simulink model "Sri_Lanka_S_FINAL"  (R2024a)
settings: Solver=VariableStepAuto  StartTime=0.0  StopTime=600  RelTol=1e-3
values from neighbouring files (symbols this model uses):
  BRO_R_P = 0.05    [FUtureGridSL.m]    (also in Sri_Lanka_FINAL.m)
  BRO_R_T = 0.38    [FUtureGridSL.m]    (also in Sri_Lanka_FINAL.m)
  BRO_T_G = 0.2    [FUtureGridSL.m]    (also in Sri_Lanka_FINAL.m)
  BRO_T_R = 5.0    (= 5)    [FUtureGridSL.m]    (also in Sri_Lanka_FINAL.m)
  BRO_T_W = 1.0    (= 1)    [FUtureGridSL.m]    (also in Sri_Lanka_FINAL.m)
  BRO_Unit_S_nom = 17.5e6    (= 17500000)    [FUtureGridSL.m]    (also in Sri_Lanka_FINAL.m)
  BWT_R_P = 0.05    [FUtureGridSL.m]    (also in Sri_Lanka.m; Sri_Lanka_FINAL.m)
  BWT_R_T = 0.38    [FUtureGridSL.m]    (also in Sri_Lanka.m; Sri_Lanka_FINAL.m)
  BWT_T_R = 5.0    (= 5)    [FUtureGridSL.m]    (also in Sri_Lanka.m; Sri_Lanka_FINAL.m)
  BWT_T_W = 1.5    [FUtureGridSL.m]    (also in Sri_Lanka.m; Sri_Lanka_FINAL.m)
  BWT_Unit_S_nom = 40e6    (= 40000000)    [FUtureGridSL.m]    (also in Sri_Lanka.m; Sri_Lanka_FINAL.m)
  CAN_R_P = 0.05    [FUtureGridSL.m]    (also in Sri_Lanka_FINAL.m)
  CAN_R_T = 0.38    [FUtureGridSL.m]    (also in Sri_Lanka_FINAL.m)
  CAN_T_G = 0.2    [FUtureGridSL.m]    (also in Sri_Lanka_FINAL.m)
  CAN_T_R = 5.0    (= 5)    [FUtureGridSL.m]    (also in Sri_Lanka_FINAL.m)
  CAN_T_W = 1.0    (= 1)    [FUtureGridSL.m]    (also in Sri_Lanka_FINAL.m)
  CAN_Unit_S_nom = 30e6    (= 30000000)    [FUtureGridSL.m]    (also in Sri_Lanka_FINAL.m)
  D_T = 1500e6/S_base_sys    (= 1.5)    [FUtureGridSL.m]    (also in Sri_Lanka.m; Sri_Lanka_FINAL.m)
  f_base = 50    [FUtureGridSL.m]    (also in Sri_Lanka.m; Sri_Lanka_FINAL.m)
  H_eq = sum(Plant_H .* Plant_S_nom .* Plant_Status) / S_base_sys    [FUtureGridSL.m]    (also in Sri_Lanka.m = sum(Plant_H .* Plant_S_nom) / S_base_sys; Sri_Lanka_FINAL.m = sum(Plant_H .* Plant_S_nom) / S_base_sys)
  KEL_CC_F_GT = 0.67    [FUtureGridSL.m]    (also in Sri_Lanka.m; Sri_Lanka_FINAL.m)
  KEL_CC_F_ST = 0.33    [FUtureGridSL.m]    (also in Sri_Lanka.m; Sri_Lanka_FINAL.m)
  KEL_CC_T_HRSG = 10.0    (= 10)    [FUtureGridSL.m]    (also in Sri_Lanka.m; Sri_Lanka_FINAL.m)
  KEL_R = 0.04    [FUtureGridSL.m]    (also in Sri_Lanka.m; Sri_Lanka_FINAL.m)
  KEL_T_CH = 0.3    [FUtureGridSL.m]    (also in Sri_Lanka.m; Sri_Lanka_FINAL.m)
  KEL_UNIT1_S_nom = 20e6    (= 20000000)    [FUtureGridSL.m]    (also in Sri_Lanka.m; Sri_Lanka_FINAL.m)
  KEL_UNIT2_S_nom = 115e6    (= 115000000)    [FUtureGridSL.m]    (also in Sri_Lanka.m; Sri_Lanka_FINAL.m)
  KEL_UNIT3_S_nom = 165e6    (= 165000000)    [FUtureGridSL.m]    (also in Sri_Lanka.m; Sri_Lanka_FINAL.m)
  KUK_R_P = 0.05    [FUtureGridSL.m]    (also in Sri_Lanka_FINAL.m)
  KUK_R_T = 0.38    [FUtureGridSL.m]    (also in Sri_Lanka_FINAL.m)
  KUK_T_R = 5.0    (= 5)    [FUtureGridSL.m]    (also in Sri_Lanka_FINAL.m)
  KUK_T_W = 0.8    [FUtureGridSL.m]    (also in Sri_Lanka_FINAL.m)
  KUK_Unit_S_nom = 40e6    (= 40000000)    [FUtureGridSL.m]    (also in Sri_Lanka_FINAL.m)
  LAK_R = 0.04    [FUtureGridSL.m]    (also in Sri_Lanka.m; Sri_Lanka_FINAL.m)
  LAK_S_nom = 300e6    (= 300000000)    [FUtureGridSL.m]    (also in Sri_Lanka.m; Sri_Lanka_FINAL.m)
  MAN_K_vir = 12.0    (= 12)    [FUtureGridSL.m]    (also in Sri_Lanka_FINAL.m)
  MAN_T_FILT = 0.02    [FUtureGridSL.m]    (also in Sri_Lanka_FINAL.m)
  MAN_T_INV = 0.05    [FUtureGridSL.m]    (also in Sri_Lanka_FINAL.m)
  MAN_Unit_S_nom = 100e6    (= 100000000)    [FUtureGridSL.m]    (also in Sri_Lanka_FINAL.m)
  NLX_R_P = 0.05    [FUtureGridSL.m]    (also in Sri_Lanka_FINAL.m)
  NLX_R_T = 0.40    (= 0.4)    [FUtureGridSL.m]    (also in Sri_Lanka_FINAL.m)
  NLX_T_G = 0.2    [FUtureGridSL.m]    (also in Sri_Lanka_FINAL.m)
  NLX_T_R = 5.0    (= 5)    [FUtureGridSL.m]    (also in Sri_Lanka_FINAL.m)
  NLX_T_W = 1.2    [FUtureGridSL.m]    (also in Sri_Lanka_FINAL.m)
  NLX_Unit_S_nom = 50e6    (= 50000000)    [FUtureGridSL.m]    (also in Sri_Lanka_FINAL.m)
  OLX_R_P = 0.05    [FUtureGridSL.m]    (also in Sri_Lanka_FINAL.m)
  OLX_R_T = 0.38    [FUtureGridSL.m]    (also in Sri_Lanka_FINAL.m)
  OLX_T_G = 0.2    [FUtureGridSL.m]    (also in Sri_Lanka_FINAL.m)
  OLX_T_R = 5.0    (= 5)    [FUtureGridSL.m]    (also in Sri_Lanka_FINAL.m)
  OLX_T_W = 1.0    (= 1)    [FUtureGridSL.m]    (also in Sri_Lanka_FINAL.m)
  OLX_Unit_S_nom_1 = 12.5e6    (= 12500000)    [FUtureGridSL.m]    (also in Sri_Lanka_FINAL.m)
  OLX_Unit_S_nom_2 = 8.33e6    (= 8330000)    [FUtureGridSL.m]    (also in Sri_Lanka_FINAL.m)
  POL_R_P = 0.05    [FUtureGridSL.m]    (also in Sri_Lanka_FINAL.m)
  POL_R_T = 0.40    (= 0.4)    [FUtureGridSL.m]    (also in Sri_Lanka_FINAL.m)
  POL_T_G = 0.2    [FUtureGridSL.m]    (also in Sri_Lanka_FINAL.m)
  POL_T_R = 5.0    (= 5)    [FUtureGridSL.m]    (also in Sri_Lanka_FINAL.m)
  POL_T_W = 1.4    [FUtureGridSL.m]    (also in Sri_Lanka_FINAL.m)
  POL_Unit_S_nom = 45e6    (= 45000000)    [FUtureGridSL.m]    (also in Sri_Lanka_FINAL.m)
  RAN_R_P = 0.05    [FUtureGridSL.m]    (also in Sri_Lanka.m; Sri_Lanka_FINAL.m)
  RAN_R_T = 0.38    [FUtureGridSL.m]    (also in Sri_Lanka.m; Sri_Lanka_FINAL.m)
  RAN_T_R = 5.0    (= 5)    [FUtureGridSL.m]    (also in Sri_Lanka.m; Sri_Lanka_FINAL.m)
  RAN_T_W = 1.2    [FUtureGridSL.m]    (also in Sri_Lanka.m; Sri_Lanka_FINAL.m)
  RAN_Unit_S_nom = 63e6    (= 63000000)    [FUtureGridSL.m]    (also in Sri_Lanka.m; Sri_Lanka_FINAL.m)
  RHT_F_HP = 0.3    [FUtureGridSL.m]    (also in Sri_Lanka.m; Sri_Lanka_FINAL.m)
  RHT_T_CH = 0.3    [FUtureGridSL.m]    (also in Sri_Lanka.m; Sri_Lanka_FINAL.m)
  RHT_T_RH = 7.0    (= 7)    [FUtureGridSL.m]    (also in Sri_Lanka.m; Sri_Lanka_FINAL.m)
  rocof_meas_window = 0.18    [FUtureGridSL.m]    (also in Sri_Lanka.m; Sri_Lanka_FINAL.m)
  RTB_R_P = 0.05    [FUtureGridSL.m]    (also in Sri_Lanka.m; Sri_Lanka_FINAL.m)
  RTB_R_T = 0.38    [FUtureGridSL.m]    (also in Sri_Lanka.m; Sri_Lanka_FINAL.m)
  RTB_T_R = 5.0    (= 5)    [FUtureGridSL.m]    (also in Sri_Lanka.m; Sri_Lanka_FINAL.m)
  RTB_T_W = 1.0    (= 1)    [FUtureGridSL.m]    (also in Sri_Lanka.m; Sri_Lanka_FINAL.m)
  RTB_Unit_S_nom = 26e6    (= 26000000)    [FUtureGridSL.m]    (also in Sri_Lanka.m; Sri_Lanka_FINAL.m)
  S_base_sys = 1000e6    (= 1000000000)    [FUtureGridSL.m]    (also in Sri_Lanka.m; Sri_Lanka_FINAL.m)
  SAM_R_P = 0.05    [FUtureGridSL.m]    (also in Sri_Lanka.m; Sri_Lanka_FINAL.m)
  SAM_R_T = 0.38    [FUtureGridSL.m]    (also in Sri_Lanka.m; Sri_Lanka_FINAL.m)
  SAM_T_R = 5.0    (= 5)    [FUtureGridSL.m]    (also in Sri_Lanka.m; Sri_Lanka_FINAL.m)
  SAM_T_W = 1.5    [FUtureGridSL.m]    (also in Sri_Lanka.m; Sri_Lanka_FINAL.m)
  SAM_Unit_S_nom = 60e6    (= 60000000)    [FUtureGridSL.m]    (also in Sri_Lanka.m; Sri_Lanka_FINAL.m)
  SOBA_GT_R = 0.04    [FUtureGridSL.m]    (also in Sri_Lanka_FINAL.m)
  SOBA_GT_S_nom = 220e6    (= 220000000)    [FUtureGridSL.m]    (also in Sri_Lanka_FINAL.m)
  SOBA_GT_T_g = 0.05    [FUtureGridSL.m]    (also in Sri_Lanka_FINAL.m)
  SOBA_GT_T_t = 0.2    [FUtureGridSL.m]    (also in Sri_Lanka_FINAL.m)
  SOBA_ST_R = 0.04    [FUtureGridSL.m]    (also in Sri_Lanka_FINAL.m)
  SOBA_ST_S_nom = 130e6    (= 130000000)    [FUtureGridSL.m]    (also in Sri_Lanka_FINAL.m)
  SOBA_ST_T_ch = 0.5    [FUtureGridSL.m]    (also in Sri_Lanka_FINAL.m)
  SOBA_ST_T_hrsga = 10.0    (= 10)    [FUtureGridSL.m]    (also in Sri_Lanka_FINAL.m)
  t_dist = 200    [FUtureGridSL.m]    (also in Sri_Lanka.m; Sri_Lanka_FINAL.m)
  T_G = 0.2    [FUtureGridSL.m]    (also in Sri_Lanka.m; Sri_Lanka_FINAL.m)
  UKU_R_P = 0.05    [FUtureGridSL.m]    (also in Sri_Lanka.m; Sri_Lanka_FINAL.m)
  UKU_R_T = 0.38    [FUtureGridSL.m]    (also in Sri_Lanka.m; Sri_Lanka_FINAL.m)
  UKU_T_R = 5.0    (= 5)    [FUtureGridSL.m]    (also in Sri_Lanka.m; Sri_Lanka_FINAL.m)
  UKU_T_W = 1.2    [FUtureGridSL.m]    (also in Sri_Lanka.m; Sri_Lanka_FINAL.m)
  UKU_Unit_S_nom = 20e6    (= 20000000)    [FUtureGridSL.m]    (also in Sri_Lanka.m; Sri_Lanka_FINAL.m)
  UMA_R_P = 0.05    [FUtureGridSL.m]    (also in Sri_Lanka_FINAL.m)
  UMA_R_T = 0.38    [FUtureGridSL.m]    (also in Sri_Lanka_FINAL.m)
  UMA_T_R = 5.0    (= 5)    [FUtureGridSL.m]    (also in Sri_Lanka_FINAL.m)
  UMA_T_W = 1.5    [FUtureGridSL.m]    (also in Sri_Lanka_FINAL.m)
  UMA_Unit_S_nom = 60e6    (= 60000000)    [FUtureGridSL.m]    (also in Sri_Lanka_FINAL.m)
  UTH_R = 0.04    [FUtureGridSL.m]    (also in Sri_Lanka.m; Sri_Lanka_FINAL.m)
  UTH_T_ACT = 0.1    [FUtureGridSL.m]    (also in Sri_Lanka.m; Sri_Lanka_FINAL.m)
  UTH_Unit_S_nom = 8e6    (= 8000000)    [FUtureGridSL.m]    (also in Sri_Lanka.m; Sri_Lanka_FINAL.m)
  WIM_R_P = 0.05    [FUtureGridSL.m]    (also in Sri_Lanka_FINAL.m)
  WIM_R_T = 0.38    [FUtureGridSL.m]    (also in Sri_Lanka_FINAL.m)
  WIM_T_G = 0.2    [FUtureGridSL.m]    (also in Sri_Lanka_FINAL.m)
  WIM_T_R = 5.0    (= 5)    [FUtureGridSL.m]    (also in Sri_Lanka_FINAL.m)
  WIM_T_W = 1.0    (= 1)    [FUtureGridSL.m]    (also in Sri_Lanka_FINAL.m)
  WIM_Unit_S_nom = 25e6    (= 25000000)    [FUtureGridSL.m]    (also in Sri_Lanka_FINAL.m)
  YUGA_GT_R = 0.04    [FUtureGridSL.m]    (also in Sri_Lanka_FINAL.m)
  YUGA_GT_S_nom = 100e6    (= 100000000)    [FUtureGridSL.m]    (also in Sri_Lanka_FINAL.m)
  YUGA_GT_T_G = 0.1    [FUtureGridSL.m]    (also in Sri_Lanka_FINAL.m)
  YUGA_GT_T_t = 0.4    [FUtureGridSL.m]    (also in Sri_Lanka_FINAL.m)
  YUGA_ST_R = 0.04    [FUtureGridSL.m]    (also in Sri_Lanka_FINAL.m)
  YUGA_ST_S_nom = 100e6    (= 100000000)    [FUtureGridSL.m]    (also in Sri_Lanka_FINAL.m)
  YUGA_ST_T_ch = 0.3    [FUtureGridSL.m]    (also in Sri_Lanka_FINAL.m)
  YUGA_ST_T_hrsga = 15.0    (= 15)    [FUtureGridSL.m]    (also in Sri_Lanka_FINAL.m)
settings Model: Creator=munas  LastModifiedBy=munas

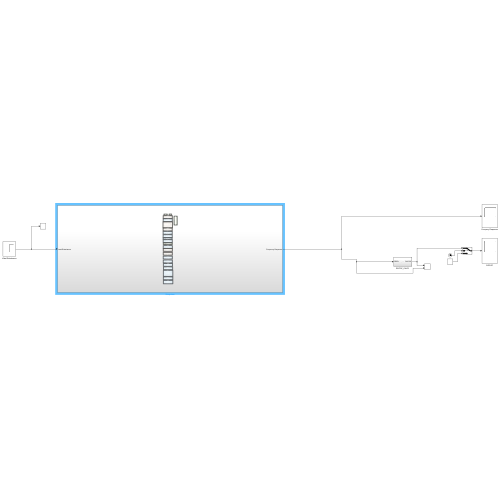
[thumbnail: Simulink's stored preview of the top-level diagram]
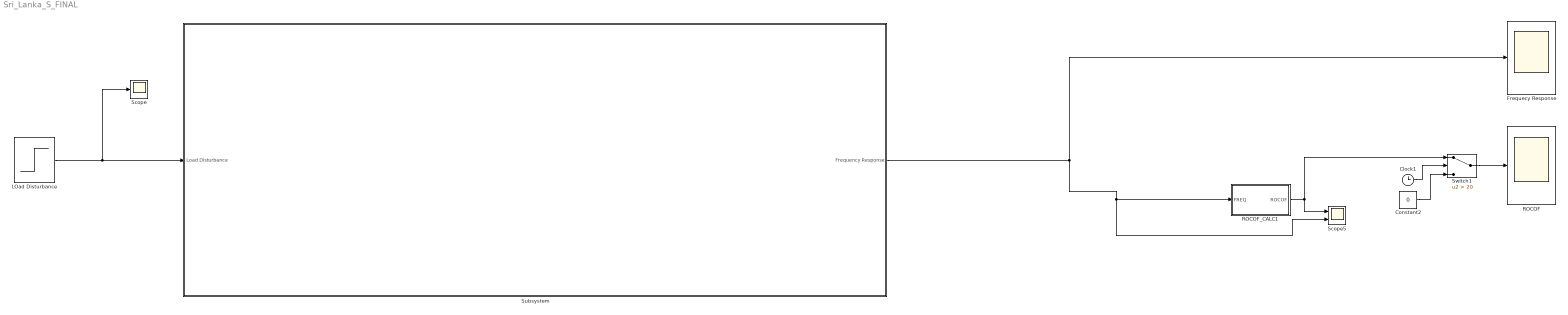
== system Sri_Lanka_S_FINAL ==
  Clock1 : Clock
  Constant2 : Constant  Value=0
  Frequecy Response : Scope
  LOad Disturbance : Step  Time=t_dist  After=0.05  SampleTime=0
  ROCOF : Scope
  ROCOF_CALC1 : Subsystem
  Scope : Scope
  Scope5 : Scope  NumInputPorts=2
  Subsystem : Subsystem
  Switch1 : Switch  Criteria=u2 > Threshold  Threshold=20  SaturateOnIntegerOverflow=off  InputSameDT=off
  wires:
  LOad Disturbance/1 -> Subsystem/1(Load Disturbance), Scope/1
  Subsystem/1(Frequency Response) -> Scope5/2, ROCOF_CALC1/1(FREQ), Frequecy Response/1
  Constant2/1 -> Switch1/3
  Switch1/1 -> ROCOF/1
  Clock1/1 -> Switch1/2
  ROCOF_CALC1/1(ROCOF) -> Switch1/1, Scope5/1

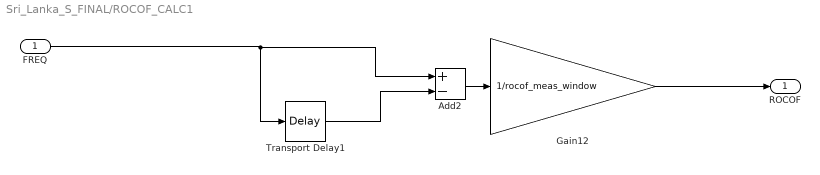
== system Sri_Lanka_S_FINAL/ROCOF_CALC1 ==
  FREQ : Inport
  Add2 : Sum  Inputs=+-
  Gain12 : Gain  Gain=1/rocof_meas_window
  Transport Delay1 : TransportDelay  DelayTime=rocof_meas_window  InitialOutput=50
  ROCOF : Outport
  wires:
  Transport Delay1/1 -> Add2/2
  Gain12/1 -> ROCOF/1
  Add2/1 -> Gain12/1
  FREQ/1 -> Add2/1, Transport Delay1/1

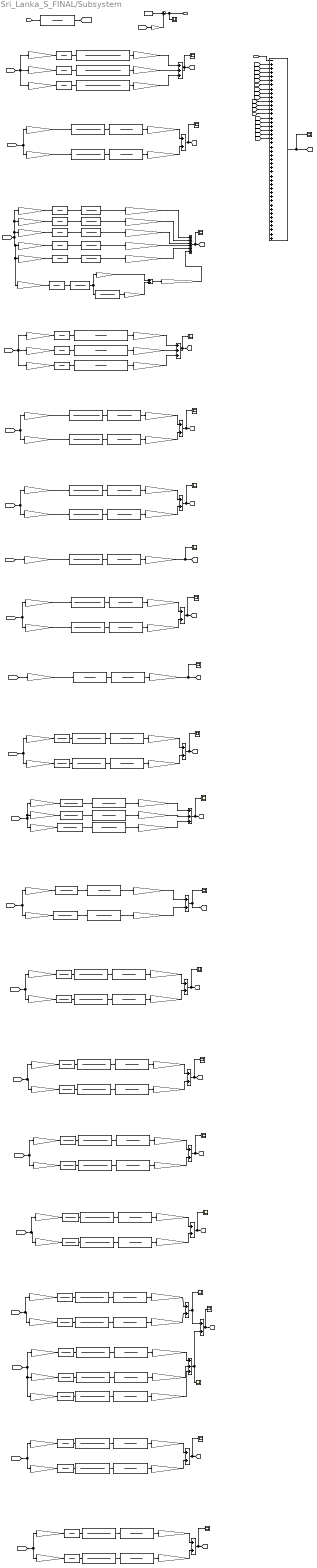
== system Sri_Lanka_S_FINAL/Subsystem ==
  note: NAYANAJITH
  note: Dinitha
  note: [Steam Turbine Path: 33%]
  note: [Gas Turbine Path: 67%]
  note: SAMANALAWEWA (60MW *2 )
  note: GRID BLOCK
  note: SUMMING BLOCK
  note: To convert to the frequency
  note: LAKVIJAYA (300MW * 3)
  note: KELANITISSA
  note: Uthuru Janani plant
  note: RANDENIGALA
  note: RANTAMBE
  note: BOWATENNA
  note: UKUWELA
  note: THAMBAPAVANI WIND FARM: 100 MW
  note: Yugadhanavi GT and ST
  note: New LAXAPANA
  note: Sobadhanavi ST and GT
  note: Polpitiya Plant
  note: Canyon Plant
  note: Wimalasurendra Plant
  note: Kukuleganga Plant
  note: Uma Oya Plant
  note: Old Laxapana Plant
  note: Broadland Plant
  Load Disturbance : Inport
  " " : TransferFcn  Denominator=[2*H_eq D_T]
  Actuator Delay : TransferFcn  Denominator="[UTH_T_ACT  1]"
  Actuator Delay1 : TransferFcn  Denominator="[UTH_T_ACT  1]"
  Actuator Delay2 : TransferFcn  Denominator="[UTH_T_ACT  1]"
  Add{,4,8,13} (4 alike) : Sum  Inputs=+++
  Add1 : Sum  Inputs=-+++++++++++++++++++++++++++++++++++++++++++
  Add{2,5..7,9..12,14..19} (14 alike) : Sum
  Add3 : Sum  Inputs=++++++
  Base Scaling Gain : Gain  Gain=SAM_Unit_S_nom / S_base_sys
  Base Scaling Gain GT : Gain  Gain=YUGA_GT_S_nom / S_base_sys
  Base Scaling Gain GT1 : Gain  Gain=YUGA_GT_S_nom / S_base_sys
  Base Scaling Gain GT2 : Gain  Gain=SOBA_GT_S_nom / S_base_sys
  Base Scaling Gain1 : Gain  Gain=SAM_Unit_S_nom / S_base_sys
  Base Scaling Gain10 : Gain  Gain=RTB_Unit_S_nom / S_base_sys
  Base Scaling Gain11 : Gain  Gain=UKU_Unit_S_nom / S_base_sys
  Base Scaling Gain12 : Gain  Gain=BWT_Unit_S_nom / S_base_sys
  Base Scaling Gain13 : Gain  Gain=UKU_Unit_S_nom / S_base_sys
  Base Scaling Gain14 : Gain  Gain=MAN_Unit_S_nom / S_base_sys
  Base Scaling Gain15 : Gain  Gain=SOBA_ST_S_nom/S_base_sys
  Base Scaling Gain16 : Gain  Gain=YUGA_ST_S_nom/S_base_sys
  Base Scaling Gain17 : Gain  Gain=NLX_Unit_S_nom / S_base_sys
  Base Scaling Gain18 : Gain  Gain=NLX_Unit_S_nom / S_base_sys
  Base Scaling Gain19 : Gain  Gain=POL_Unit_S_nom / S_base_sys
  Base Scaling Gain2 : Gain  Gain=RTB_Unit_S_nom / S_base_sys
  Base Scaling Gain20 : Gain  Gain=POL_Unit_S_nom / S_base_sys
  Base Scaling Gain21 : Gain  Gain=WIM_Unit_S_nom / S_base_sys
  Base Scaling Gain22 : Gain  Gain=WIM_Unit_S_nom / S_base_sys
  Base Scaling Gain23 : Gain  Gain=BRO_Unit_S_nom / S_base_sys
  Base Scaling Gain24 : Gain  Gain=BRO_Unit_S_nom / S_base_sys
  Base Scaling Gain25 : Gain  Gain=OLX_Unit_S_nom_1 / S_base_sys
  Base Scaling Gain26 : Gain  Gain=OLX_Unit_S_nom_1 / S_base_sys
  Base Scaling Gain27 : Gain  Gain=OLX_Unit_S_nom_2 / S_base_sys
  Base Scaling Gain28 : Gain  Gain=OLX_Unit_S_nom_2 / S_base_sys
  Base Scaling Gain29 : Gain  Gain=OLX_Unit_S_nom_2 / S_base_sys
  Base Scaling Gain{3..6} (4 alike) : Gain  Gain=KEL_UNIT1_S_nom/ S_base_sys
  Base Scaling Gain30 : Gain  Gain=UMA_Unit_S_nom / S_base_sys
  Base Scaling Gain31 : Gain  Gain=UMA_Unit_S_nom / S_base_sys
  Base Scaling Gain32 : Gain  Gain=KUK_Unit_S_nom / S_base_sys
  Base Scaling Gain33 : Gain  Gain=KUK_Unit_S_nom / S_base_sys
  Base Scaling Gain34 : Gain  Gain=CAN_Unit_S_nom / S_base_sys
  Base Scaling Gain35 : Gain  Gain=CAN_Unit_S_nom / S_base_sys
  Base Scaling Gain7 : Gain  Gain=KEL_UNIT2_S_nom/ S_base_sys
  Base Scaling Gain8 : Gain  Gain=RAN_Unit_S_nom / S_base_sys
  Base Scaling Gain9 : Gain  Gain=RAN_Unit_S_nom / S_base_sys
  Combustr : TransferFcn  Denominator="[KEL_T_CH  1]"
  Constant : Constant  Value=f_base
  Gain1 : Gain  Gain=KEL_CC_F_ST
  Gain2 : Gain  Gain=KEL_UNIT3_S_nom/ S_base_sys
  Gain3 : Gain  Gain=f_base
  Governer : TransferFcn  Denominator=[T_G 1]
  Governer {1..2,7,9,11,13,15,17..19,30..33} (14 alike) : TransferFcn  Denominator=[T_G 1]
  Governer {8,10,12,14,16} (5 alike) : TransferFcn  Denominator="[KEL_T_CH  1]"
  Governer 20 : TransferFcn  Denominator=[CAN_T_G 1]
  Governer 21 : TransferFcn  Denominator="[WIM_T_G  1]"
  Governer 22 : TransferFcn  Denominator="[WIM_T_G  1]"
  Governer 23 : TransferFcn  Denominator="[BRO_T_G  1]"
  Governer 24 : TransferFcn  Denominator="[BRO_T_G  1]"
  Governer {25..29} (5 alike) : TransferFcn  Denominator="[OLX_T_G  1]"
  Governer 3 : TransferFcn  Denominator=[POL_T_G 1]
  Governer 34 : TransferFcn  Denominator="[CAN_T_G  1]"
  Governer 4 : TransferFcn  Denominator=[POL_T_G 1]
  Governer 5 : TransferFcn  Denominator=[NLX_T_G 1]
  Governer 6 : TransferFcn  Denominator=[NLX_T_G 1]
  Governer GT : TransferFcn  Denominator=[YUGA_GT_T_G 1]
  Governer GT1 : TransferFcn  Denominator=[YUGA_GT_T_G 1]
  Governer GT2 : TransferFcn  Denominator=[SOBA_GT_T_g 1]
  Governer ST : TransferFcn  Denominator=[YUGA_ST_T_ch 1]
  Governer ST1 : TransferFcn  Denominator=[SOBA_ST_T_ch 1]
  Governer1 : TransferFcn  Denominator=[T_G 1]
  HRSG Delay : TransferFcn  Denominator="[KEL_CC_T_HRSG  1]"
  Inverter Delay : TransferFcn  Denominator="[MAN_T_INV  1]"
  PURE DROOP : Gain  Gain=-1/LAK_R
  PURE DROOP GT : Gain  Gain=-1/YUGA_GT_R
  PURE DROOP GT1 : Gain  Gain=-1/YUGA_GT_R
  PURE DROOP GT2 : Gain  Gain=-1/SOBA_GT_R
  PURE DROOP ST : Gain  Gain=-1/YUGA_ST_R
  PURE DROOP ST1 : Gain  Gain=-1/SOBA_ST_R
  PURE DROOP1 : Gain  Gain=-1/LAK_R
  PURE DROOP{6..11} (6 alike) : Gain  Gain=-1/KEL_R
  PURE DROOP12 : Gain  Gain=-1/UTH_R
  PURE DROOP13 : Gain  Gain=-1/UTH_R
  PURE DROOP14 : Gain  Gain=-1/UTH_R
  PURE DROOP15 : Gain  Gain=-1/RAN_R_P
  PURE DROOP16 : Gain  Gain=-1/RAN_R_P
  PURE DROOP17 : Gain  Gain=-1/RTB_R_P
  PURE DROOP18 : Gain  Gain=-1/UKU_R_P
  PURE DROOP19 : Gain  Gain=-1/BWT_R_P
  PURE DROOP2 : Gain  Gain=-1/LAK_R
  PURE DROOP20 : Gain  Gain=-1/UKU_R_P
  PURE DROOP21 : Gain  Gain=-1/BWT_R_P
  PURE DROOP22 : Gain  Gain=-1/NLX_R_P
  PURE DROOP23 : Gain  Gain=-1/NLX_R_P
  PURE DROOP24 : Gain  Gain=-1/POL_R_P
  PURE DROOP25 : Gain  Gain=-1/POL_R_P
  PURE DROOP26 : Gain  Gain=-1/CAN_R_P
  PURE DROOP27 : Gain  Gain=-1/WIM_R_P
  PURE DROOP28 : Gain  Gain=-1/WIM_R_P
  PURE DROOP29 : Gain  Gain=-1/BRO_R_P
  PURE DROOP3 : Gain  Gain=-1/SAM_R_P
  PURE DROOP30 : Gain  Gain=-1/BRO_R_P
  PURE DROOP{31..35} (5 alike) : Gain  Gain=-1/OLX_R_P
  PURE DROOP36 : Gain  Gain=-1/UMA_R_P
  PURE DROOP37 : Gain  Gain=-1/UMA_R_P
  PURE DROOP38 : Gain  Gain=-1/KUK_R_P
  PURE DROOP39 : Gain  Gain=-1/KUK_R_P
  PURE DROOP4 : Gain  Gain=-1/SAM_R_P
  PURE DROOP40 : Gain  Gain=-1/CAN_R_P
  PURE DROOP5 : Gain  Gain=-1/RTB_R_P
  Scaling : Sum
  Scaling 1 : Gain  Gain=LAK_S_nom / S_base_sys
  Scaling 2 : Gain  Gain=LAK_S_nom / S_base_sys
  Scaling 3 : Gain  Gain=LAK_S_nom / S_base_sys
  Scaling 4 : Gain  Gain=UTH_Unit_S_nom / S_base_sys
  Scaling 5 : Gain  Gain=UTH_Unit_S_nom / S_base_sys
  Scaling 6 : Gain  Gain=UTH_Unit_S_nom / S_base_sys
  Scope{,1..22} (23 alike) : Scope
  Sum : Sum  Inputs=|++
  Synthetic Inertia : TransferFcn  Numerator="[MAN_K_vir  0]"  Denominator="[MAN_T_FILT  1]"
  Transient Droop : TransferFcn  Numerator="[SAM_T_R  1]"  Denominator="[SAM_T_R*(SAM_R_T/SAM_R_P)  1]"
  Transient Droop GT : TransferFcn  Denominator="[YUGA_GT_T_t  1]"
  Transient Droop GT1 : TransferFcn  Denominator="[YUGA_GT_T_t  1]"
  Transient Droop GT2 : TransferFcn  Denominator="[SOBA_GT_T_t  1]"
  Transient Droop ST : TransferFcn  Denominator="[YUGA_ST_T_hrsga  1]"
  Transient Droop ST1 : TransferFcn  Denominator="[SOBA_ST_T_hrsga  1]"
  Transient Droop1 : TransferFcn  Numerator="[SAM_T_R  1]"  Denominator="[SAM_T_R*(SAM_R_T/SAM_R_P)  1]"
  Transient Droop10 : TransferFcn  Numerator="[NLX_T_R  1]"  Denominator="[NLX_T_R*(NLX_R_T/NLX_R_P)  1]"
  Transient Droop11 : TransferFcn  Numerator=[POL_T_R 1]  Denominator="[POL_T_R*(POL_R_T/POL_R_P)  1]"
  Transient Droop12 : TransferFcn  Numerator="[POL_T_R  1]"  Denominator="[POL_T_R*(POL_R_T/POL_R_P)  1]"
  Transient Droop13 : TransferFcn  Numerator=[BRO_T_R 1]  Denominator="[BRO_T_R*(BRO_R_T/BRO_R_P)  1]"
  Transient Droop14 : TransferFcn  Numerator=[BRO_T_R 1]  Denominator="[BRO_T_R*(BRO_R_T/BRO_R_P)  1]"
  Transient Droop{15..19} (5 alike) : TransferFcn  Numerator=[OLX_T_R 1]  Denominator="[OLX_T_R*(OLX_R_T/OLX_R_P)  1]"
  Transient Droop2 : TransferFcn  Numerator="[RAN_T_R  1]"  Denominator="[(RAN_R_T / RAN_R_P) * RAN_T_R   1]"
  Transient Droop20 : TransferFcn  Numerator="[UMA_T_R  1]"  Denominator="[UMA_T_R*(UMA_R_T/UMA_R_P)  1]"
  Transient Droop21 : TransferFcn  Numerator="[UMA_T_R  1]"  Denominator="[UMA_T_R*(UMA_R_T/UMA_R_P)  1]"
  Transient Droop22 : TransferFcn  Numerator="[KUK_T_R  1]"  Denominator="[KUK_T_R*(KUK_R_T/KUK_R_P)  1]"
  Transient Droop23 : TransferFcn  Numerator="[KUK_T_R  1]"  Denominator="[KUK_T_R*(KUK_R_T/KUK_R_P)  1]"
  Transient Droop24 : TransferFcn  Numerator=[CAN_T_R 1]  Denominator="[CAN_T_R*(CAN_R_T/CAN_R_P)  1]"
  Transient Droop25 : TransferFcn  Numerator=[CAN_T_R 1]  Denominator="[CAN_T_R*(CAN_R_T/CAN_R_P)  1]"
  Transient Droop26 : TransferFcn  Numerator=[WIM_T_R 1]  Denominator="[WIM_T_R*(WIM_R_T/WIM_R_P)  1]"
  Transient Droop27 : TransferFcn  Numerator=[WIM_T_R 1]  Denominator="[WIM_T_R*(WIM_R_T/WIM_R_P)  1]"
  Transient Droop3 : TransferFcn  Numerator="[RAN_T_R  1]"  Denominator="[(RAN_R_T / RAN_R_P) * RAN_T_R   1]"
  Transient Droop4 : TransferFcn  Numerator="[RTB_T_R  1]"  Denominator="[(RTB_R_T / RTB_R_P) * RTB_T_R   1]"
  Transient Droop5 : TransferFcn  Numerator="[RTB_T_R  1]"  Denominator="[(RTB_R_T / RTB_R_P) * RTB_T_R   1]"
  Transient Droop6 : TransferFcn  Numerator="[BWT_T_R  1]"  Denominator="[(BWT_R_T / BWT_R_P) * BWT_T_R   1]"
  Transient Droop7 : TransferFcn  Numerator="[UKU_T_R  1]"  Denominator="[(UKU_R_T / UKU_R_P) * UKU_T_R   1]"
  Transient Droop8 : TransferFcn  Numerator="[UKU_T_R  1]"  Denominator="[(UKU_R_T / UKU_R_P) * UKU_T_R   1]"
  Transient Droop9 : TransferFcn  Numerator=[NLX_T_R 1]  Denominator="[NLX_T_R*(NLX_R_T/NLX_R_P)  1]"
  Turbine Dynamics (Reheat) : TransferFcn  Numerator="[RHT_F_HP*RHT_T_RH  1]"  Denominator="[RHT_T_CH*RHT_T_RH  (RHT_T_CH+RHT_T_RH)  1]"
  Turbine Dynamics (Reheat)1 : TransferFcn  Numerator="[RHT_F_HP*RHT_T_RH  1]"  Denominator="[RHT_T_CH*RHT_T_RH  (RHT_T_CH+RHT_T_RH)  1]"
  Turbine Dynamics (Reheat)2 : TransferFcn  Numerator="[RHT_F_HP*RHT_T_RH  1]"  Denominator="[RHT_T_CH*RHT_T_RH  (RHT_T_CH+RHT_T_RH)  1]"
  Water Column : TransferFcn  Numerator="[-SAM_T_W  1]"  Denominator="[0.5*SAM_T_W  1]"
  Water Column1 : TransferFcn  Numerator="[-SAM_T_W  1]"  Denominator="[0.5*SAM_T_W  1]"
  Water Column10 : TransferFcn  Numerator="[-NLX_T_W  1]"  Denominator="[0.5*NLX_T_W  1]"
  Water Column11 : TransferFcn  Numerator="[-POL_T_W  1]"  Denominator="[0.5*POL_T_W  1]"
  Water Column12 : TransferFcn  Numerator="[-POL_T_W  1]"  Denominator="[0.5*POL_T_W  1]"
  Water Column13 : TransferFcn  Numerator="[-BRO_T_W  1]"  Denominator="[0.5*BRO_T_W  1]"
  Water Column14 : TransferFcn  Numerator="[-BRO_T_W  1]"  Denominator="[0.5*BRO_T_W  1]"
  Water Column{15..19} (5 alike) : TransferFcn  Numerator="[-OLX_T_W  1]"  Denominator="[0.5*OLX_T_W  1]"
  Water Column2 : TransferFcn  Numerator="[-RAN_T_W  1]"  Denominator="[0.5 * RAN_T_W   1]"
  Water Column20 : TransferFcn  Numerator="[-UMA_T_W  1]"  Denominator="[0.5*UMA_T_W  1]"
  Water Column21 : TransferFcn  Numerator="[-UMA_T_W  1]"  Denominator="[0.5*UMA_T_W  1]"
  Water Column22 : TransferFcn  Numerator="[-KUK_T_W  1]"  Denominator="[0.5*KUK_T_W  1]"
  Water Column23 : TransferFcn  Numerator="[-KUK_T_W  1]"  Denominator="[0.5*KUK_T_W  1]"
  Water Column24 : TransferFcn  Numerator="[-CAN_T_W  1]"  Denominator="[0.5*CAN_T_W  1]"
  Water Column25 : TransferFcn  Numerator="[-CAN_T_W  1]"  Denominator="[0.5*CAN_T_W  1]"
  Water Column26 : TransferFcn  Numerator="[-WIM_T_W  1]"  Denominator="[0.5*WIM_T_W  1]"
  Water Column27 : TransferFcn  Numerator="[-WIM_T_W  1]"  Denominator="[0.5*WIM_T_W  1]"
  Water Column3 : TransferFcn  Numerator="[-RAN_T_W  1]"  Denominator="[0.5 * RAN_T_W   1]"
  Water Column4 : TransferFcn  Numerator="[-RTB_T_W  1]"  Denominator="[0.5 * RTB_T_W   1]"
  Water Column5 : TransferFcn  Numerator="[-RTB_T_W  1]"  Denominator="[0.5 * RTB_T_W   1]"
  Water Column6 : TransferFcn  Numerator="[-BWT_T_W  1]"  Denominator="[0.5 * BWT_T_W   1]"
  Water Column7 : TransferFcn  Numerator="[-UKU_T_W  1]"  Denominator="[0.5 * UKU_T_W   1]"
  Water Column8 : TransferFcn  Numerator="[-UKU_T_W  1]"  Denominator="[0.5 * UKU_T_W   1]"
  Water Column9 : TransferFcn  Numerator="[-NLX_T_W  1]"  Denominator="[0.5*NLX_T_W  1]"
  | Gain: F_GT : Gain  Gain=KEL_CC_F_GT
  Frequency Response : Outport
  wires:
  Governer 1/1 -> Turbine Dynamics (Reheat)/1
  Turbine Dynamics (Reheat)/1 -> Scaling 1/1
  PURE DROOP/1 -> Governer 1/1
  Sum/1 -> Scope2/1, Frequency Response/1
  Constant/1 -> Sum/1
  Scaling 1/1 -> Add/1
  PURE DROOP1/1 -> Governer 2/1
  Governer 2/1 -> Turbine Dynamics (Reheat)1/1
  Turbine Dynamics (Reheat)1/1 -> Scaling 2/1
  Scaling 2/1 -> Add/2
  Governer/1 -> Turbine Dynamics (Reheat)2/1
  PURE DROOP2/1 -> Governer/1
  Turbine Dynamics (Reheat)2/1 -> Scaling 3/1
  Scaling 3/1 -> Add/3
  Add/1 -> Scope3/1, [LAK]
  [P_acc] -> " "/1
  " "/1 -> [Rotor_Dev]
  [Rotor_Dev] -> PURE DROOP2/1, PURE DROOP/1, PURE DROOP1/1
  [Rotor_Dev] -> Gain3/1
  [LAK] -> Add1/2
  Add1/1 -> Scope/1, [P_acc]
  Load Disturbance/1 -> Add1/1
  [Rotor_Dev] -> PURE DROOP4/1, PURE DROOP3/1
  Base Scaling Gain/1 -> Add2/1
  PURE DROOP3/1 -> Transient Droop/1
  Add2/1 -> Scope1/1, [SAM]
  Transient Droop/1 -> Water Column/1
  Water Column/1 -> Base Scaling Gain/1
  Water Column1/1 -> Base Scaling Gain1/1
  Transient Droop1/1 -> Water Column1/1
  PURE DROOP4/1 -> Transient Droop1/1
  Base Scaling Gain1/1 -> Add2/2
  [SAM] -> Add1/3
  Gain3/1 -> Sum/2
  [Rotor_Dev] -> PURE DROOP8/1, PURE DROOP7/1, PURE DROOP6/1, PURE DROOP11/1, PURE DROOP10/1, PURE DROOP9/1
  Governer 7/1 -> Governer 8/1
  PURE DROOP6/1 -> Governer 7/1
  Governer 8/1 -> Base Scaling Gain3/1
  Governer 9/1 -> Governer 10/1
  PURE DROOP7/1 -> Governer 9/1
  Governer 10/1 -> Base Scaling Gain4/1
  Governer 11/1 -> Governer 12/1
  PURE DROOP8/1 -> Governer 11/1
  Governer 12/1 -> Base Scaling Gain5/1
  Governer 13/1 -> Governer 14/1
  PURE DROOP9/1 -> Governer 13/1
  Governer 14/1 -> Base Scaling Gain6/1
  Governer 15/1 -> Governer 16/1
  PURE DROOP10/1 -> Governer 15/1
  Governer 16/1 -> Base Scaling Gain7/1
  PURE DROOP11/1 -> Governer 17/1
  Governer 17/1 -> Combustr/1
  HRSG Delay/1 -> Gain1/1
  Combustr/1 -> HRSG Delay/1, | Gain: F_GT/1
  | Gain: F_GT/1 -> Scaling/1
  Gain1/1 -> Scaling/2
  Scaling/1 -> Gain2/1
  Base Scaling Gain3/1 -> Add3/1
  Base Scaling Gain4/1 -> Add3/2
  Base Scaling Gain5/1 -> Add3/3
  Base Scaling Gain6/1 -> Add3/4
  Base Scaling Gain7/1 -> Add3/5
  Gain2/1 -> Add3/6
  Add3/1 -> Scope9/1, [KEL]
  [KEL] -> Add1/4
  Actuator Delay2/1 -> Scaling 6/1
  PURE DROOP13/1 -> Governer 19/1
  PURE DROOP12/1 -> Governer 18/1
  PURE DROOP14/1 -> Governer1/1
  Add4/1 -> Scope4/1, [UTH]
  Scaling 6/1 -> Add4/3
  Governer 19/1 -> Actuator Delay1/1
  Governer1/1 -> Actuator Delay2/1
  Scaling 4/1 -> Add4/1
  [Rotor_Dev] -> PURE DROOP14/1, PURE DROOP12/1, PURE DROOP13/1
  Actuator Delay1/1 -> Scaling 5/1
  Governer 18/1 -> Actuator Delay/1
  Scaling 5/1 -> Add4/2
  Actuator Delay/1 -> Scaling 4/1
  [UTH] -> Add1/5
  [Rotor_Dev] -> PURE DROOP16/1, PURE DROOP15/1
  Transient Droop2/1 -> Water Column2/1
  Base Scaling Gain8/1 -> Add5/1
  Water Column2/1 -> Base Scaling Gain8/1
  Add5/1 -> Scope5/1, [RAN]
  Transient Droop3/1 -> Water Column3/1
  Water Column3/1 -> Base Scaling Gain9/1
  Base Scaling Gain9/1 -> Add5/2
  [RAN] -> Add1/6
  PURE DROOP5/1 -> Transient Droop4/1
  Add6/1 -> Scope6/1, [RTB]
  [Rotor_Dev] -> PURE DROOP17/1, PURE DROOP5/1
  Water Column4/1 -> Base Scaling Gain2/1
  Base Scaling Gain2/1 -> Add6/1
  Base Scaling Gain10/1 -> Add6/2
  Transient Droop4/1 -> Water Column4/1
  [RTB] -> Add1/7
  PURE DROOP15/1 -> Transient Droop2/1
  PURE DROOP16/1 -> Transient Droop3/1
  Transient Droop5/1 -> Water Column5/1
  PURE DROOP17/1 -> Transient Droop5/1
  Water Column5/1 -> Base Scaling Gain10/1
  PURE DROOP19/1 -> Transient Droop6/1
  Transient Droop6/1 -> Water Column6/1
  [Rotor_Dev] -> PURE DROOP19/1
  Water Column6/1 -> Base Scaling Gain12/1
  Base Scaling Gain12/1 -> Scope7/1, [BWT]
  [BWT] -> Add1/8
  PURE DROOP20/1 -> Transient Droop7/1
  Transient Droop7/1 -> Water Column7/1
  Base Scaling Gain13/1 -> Add7/1
  [Rotor_Dev] -> PURE DROOP18/1, PURE DROOP20/1
  Water Column7/1 -> Base Scaling Gain13/1
  Add7/1 -> Scope8/1, [UKU]
  Base Scaling Gain11/1 -> Add7/2
  Water Column8/1 -> Base Scaling Gain11/1
  Transient Droop8/1 -> Water Column8/1
  PURE DROOP18/1 -> Transient Droop8/1
  [UKU] -> Add1/9
  Base Scaling Gain14/1 -> Scope10/1, [MAN]
  Inverter Delay/1 -> Base Scaling Gain14/1
  [Rotor_Dev] -> PURE DROOP21/1
  PURE DROOP21/1 -> Synthetic Inertia/1
  Synthetic Inertia/1 -> Inverter Delay/1
  [MAN] -> Add1/10
  Water Column10/1 -> Base Scaling Gain18/1
  Water Column11/1 -> Base Scaling Gain19/1
  PURE DROOP23/1 -> Governer 6/1
  Governer 6/1 -> Transient Droop10/1
  Base Scaling Gain GT2/1 -> Add9/1
  Base Scaling Gain17/1 -> Add10/1
  Transient Droop10/1 -> Water Column10/1
  Governer GT2/1 -> Transient Droop GT2/1
  Add9/1 -> Scope12/1, [SOBA]
  Transient Droop9/1 -> Water Column9/1
  PURE DROOP GT2/1 -> Governer GT2/1
  Base Scaling Gain GT/1 -> Add8/1
  Base Scaling Gain15/1 -> Add9/2
  Governer ST/1 -> Transient Droop ST/1
  Transient Droop GT/1 -> Base Scaling Gain GT/1
  [Rotor_Dev] -> PURE DROOP ST/1, PURE DROOP GT1/1, PURE DROOP GT/1
  Base Scaling Gain GT1/1 -> Add8/2
  Transient Droop GT1/1 -> Base Scaling Gain GT1/1
  Governer 3/1 -> Transient Droop11/1
  [Rotor_Dev] -> PURE DROOP25/1, PURE DROOP24/1
  Governer 5/1 -> Transient Droop9/1
  PURE DROOP25/1 -> Governer 4/1
  Base Scaling Gain19/1 -> Add11/1
  Base Scaling Gain18/1 -> Add10/2
  Transient Droop GT2/1 -> Base Scaling Gain GT2/1
  Governer GT/1 -> Transient Droop GT/1
  Add8/1 -> Scope11/1, [YUGA]
  Transient Droop ST/1 -> Base Scaling Gain16/1
  Governer 4/1 -> Transient Droop12/1
  [Rotor_Dev] -> PURE DROOP23/1, PURE DROOP22/1
  [Rotor_Dev] -> PURE DROOP ST1/1, PURE DROOP GT2/1
  Add11/1 -> Scope14/1, [POL]
  PURE DROOP ST/1 -> Governer ST/1
  PURE DROOP ST1/1 -> Governer ST1/1
  Base Scaling Gain20/1 -> Add11/2
  PURE DROOP GT/1 -> Governer GT/1
  Transient Droop ST1/1 -> Base Scaling Gain15/1
  Transient Droop11/1 -> Water Column11/1
  PURE DROOP22/1 -> Governer 5/1
  Governer GT1/1 -> Transient Droop GT1/1
  Base Scaling Gain16/1 -> Add8/3
  Add10/1 -> Scope13/1, [NLX]
  Water Column9/1 -> Base Scaling Gain17/1
  PURE DROOP24/1 -> Governer 3/1
  Water Column12/1 -> Base Scaling Gain20/1
  Governer ST1/1 -> Transient Droop ST1/1
  Transient Droop12/1 -> Water Column12/1
  PURE DROOP GT1/1 -> Governer GT1/1
  [NLX] -> Add1/13
  [YUGA] -> Add1/12
  [SOBA] -> Add1/11
  [POL] -> Add1/14
  Base Scaling Gain33/1 -> Add16/2
  Transient Droop21/1 -> Water Column21/1
  Add14/1 -> Scope18/1, [OLX]
  Governer 29/1 -> Transient Droop19/1
  PURE DROOP28/1 -> Governer 22/1
  [Rotor_Dev] -> PURE DROOP39/1, PURE DROOP38/1
  Base Scaling Gain21/1 -> Add18/1
  Governer 27/1 -> Transient Droop18/1
  Base Scaling Gain24/1 -> Add19/2
  Governer 33/1 -> Transient Droop23/1
  PURE DROOP33/1 -> Governer 27/1
  Base Scaling Gain32/1 -> Add16/1
  PURE DROOP38/1 -> Governer 32/1
  Transient Droop20/1 -> Water Column20/1
  Water Column15/1 -> Base Scaling Gain25/1
  Water Column23/1 -> Base Scaling Gain33/1
  Base Scaling Gain31/1 -> Add15/2
  PURE DROOP29/1 -> Governer 23/1
  Governer 26/1 -> Transient Droop15/1
  PURE DROOP35/1 -> Governer 29/1
  Base Scaling Gain30/1 -> Add15/1
  Water Column21/1 -> Base Scaling Gain31/1
  PURE DROOP37/1 -> Governer 31/1
  Base Scaling Gain28/1 -> Add13/2
  Add15/1 -> Scope19/1, [UMA]
  Governer 30/1 -> Transient Droop20/1
  PURE DROOP36/1 -> Governer 30/1
  [Rotor_Dev] -> PURE DROOP31/1, PURE DROOP32/1
  Water Column13/1 -> Base Scaling Gain23/1
  Governer 28/1 -> Transient Droop17/1
  [Rotor_Dev] -> PURE DROOP26/1, PURE DROOP40/1
  [Rotor_Dev] -> PURE DROOP29/1, PURE DROOP30/1
  Transient Droop19/1 -> Water Column19/1
  Add18/1 -> Scope22/1, [WIM]
  Water Column18/1 -> Base Scaling Gain28/1
  Add13/1 -> Add14/2, Scope17/1
  Water Column22/1 -> Base Scaling Gain32/1
  Transient Droop14/1 -> Water Column14/1
  Governer 24/1 -> Transient Droop13/1
  Transient Droop15/1 -> Water Column15/1
  Base Scaling Gain27/1 -> Add13/1
  [Rotor_Dev] -> PURE DROOP35/1, PURE DROOP33/1, PURE DROOP34/1
  Water Column24/1 -> Base Scaling Gain34/1
  Transient Droop22/1 -> Water Column22/1
  Water Column16/1 -> Base Scaling Gain26/1
  Transient Droop18/1 -> Water Column18/1
  Governer 25/1 -> Transient Droop16/1
  Transient Droop17/1 -> Water Column17/1
  Water Column14/1 -> Base Scaling Gain24/1
  PURE DROOP32/1 -> Governer 26/1
  Base Scaling Gain22/1 -> Add18/2
  [Rotor_Dev] -> PURE DROOP27/1, PURE DROOP28/1
  PURE DROOP30/1 -> Governer 24/1
  Governer 21/1 -> Transient Droop27/1
  Transient Droop16/1 -> Water Column16/1
  Base Scaling Gain29/1 -> Add13/3
  Transient Droop26/1 -> Water Column26/1
  Governer 23/1 -> Transient Droop14/1
  Transient Droop27/1 -> Water Column27/1
  PURE DROOP34/1 -> Governer 28/1
  [Rotor_Dev] -> PURE DROOP37/1, PURE DROOP36/1
  PURE DROOP27/1 -> Governer 21/1
  Base Scaling Gain23/1 -> Add19/1
  Transient Droop13/1 -> Water Column13/1
  Water Column25/1 -> Base Scaling Gain35/1
  Governer 20/1 -> Transient Droop25/1
  Add19/1 -> Scope15/1, [BRO]
  PURE DROOP26/1 -> Governer 20/1
  Transient Droop25/1 -> Water Column25/1
  Water Column17/1 -> Base Scaling Gain27/1
  Base Scaling Gain34/1 -> Add17/1
  Governer 34/1 -> Transient Droop24/1
  Transient Droop24/1 -> Water Column24/1
  Governer 22/1 -> Transient Droop26/1
  Base Scaling Gain26/1 -> Add12/2
  PURE DROOP40/1 -> Governer 34/1
  Add16/1 -> Scope20/1, [KUK]
  Base Scaling Gain35/1 -> Add17/2
  Water Column26/1 -> Base Scaling Gain21/1
  Add17/1 -> Scope21/1, [CAN]
  PURE DROOP39/1 -> Governer 33/1
  Add12/1 -> Add14/1, Scope16/1
  Governer 32/1 -> Transient Droop22/1
  Governer 31/1 -> Transient Droop21/1
  Water Column27/1 -> Base Scaling Gain22/1
  Water Column20/1 -> Base Scaling Gain30/1
  Transient Droop23/1 -> Water Column23/1
  PURE DROOP31/1 -> Governer 25/1
  Water Column19/1 -> Base Scaling Gain29/1
  Base Scaling Gain25/1 -> Add12/1
  [BRO] -> Add1/17
  [WIM] -> Add1/16
  [UMA] -> Add1/19
  [CAN] -> Add1/15
  [KUK] -> Add1/20
  [OLX] -> Add1/18
